simulink model "gm_flyback_pid"  (R2021b)
settings: Solver=FixedStepDiscrete  StartTime=0.0  StopTime=100e-3  RelTol=1e-3
undefined symbols (not defined in the file or in its folder): DiscIntNeverNeededParam
Description:
  | Symmetric FIR Filter
  | This example shows how to use HDL Coder(TM) to check, generate,
  | and verify HDL for a fixed-point symmetric FIR filter.
settings Model: Creator=The MathWorks, Inc.  LastModifiedBy=Marco Milanesi
settings SolverCC: AlgebraicLoopSolver=TrustRegion  AutoInsertRateTranBlk=on
settings DataIOCC: LimitDataPoints=on  SaveFormat=Array  SaveOutput=off  SignalLogging=off  SaveTime=off  ReturnWorkspaceOutputs=off  SignalLoggingName=logsOut
settings OptimizationCC: BlockReduction=off  BooleanDataType=off  ConditionallyExecuteInputs=off  DefaultParameterBehavior=Inlined  InheritOutputTypeSmallerThanSingle=on  InlineInvariantSignals=on  ExpressionDepthLimit=2147483647  InitFltsAndDblsToZero=on  LifeSpan=inf  BufferReusableBoundary=off
settings DebuggingCC: AlgebraicLoopMsg=error  SaveWithParameterizedLinksMsg=none  UnderspecifiedInitializationDetection=Classic  MergeDetectMultiDrivingBlocksExec=none  CheckExecutionContextPreStartOutputMsg=on  SignalResolutionControl=TryResolveAllWithWarning  InheritedTsInSrcMsg=none  MultiTaskDSMMsg=warning  MultiTaskCondExecSysMsg=none  SingleTaskRateTransMsg=error  IntegerOverflowMsg=none  ParameterPrecisionLossMsg=none  FcnCallInpInsideContextMsg=warning  BusObjectLabelMismatch=none  StateNameClashWarn=warning  SFUnexpectedBacktrackingDiag=warning  SFNoUnconditionalDefaultTransitionDiag=warning  SFExecutionAtInitializationDiag=none  SFMachineParentedDataDiag=warning  IntegerSaturationMsg=none  ArithmeticOperatorsInVariantConditions=warning
settings HardwareCC: ProdBitPerPointer=32  ProdBitPerSizeT=32  ProdBitPerPtrDiffT=32  ProdLargestAtomicFloat=None  ProdIntDivRoundTo=Undefined  ProdEndianess=Unspecified  ProdWordSize=32  ProdHWDeviceType=ASIC/FPGA  TargetUnknown=on  ProdEqTarget=off
settings ModelReferenceCC: PropagateSignalLabelsOutOfModel=off
settings SFSimCC: SimUseLocalCustomCode=off  CustomCodeUndefinedFunction=UseInterfaceOnly
settings RTWCC: RTWUseLocalCustomCode=off
settings CodeAppCC: StateflowObjectComments=on
settings GRTTargetCC: TargetFcnLib=ansi_tfl_tmw.mat  TargetLangStandard=C89/C90 (ANSI)  CombineOutputUpdateFcns=off  GRTInterface=on
settings ConfigComp: CovMetricSettings=dw  CovSaveCumulativeToWorkspaceVar=on  CovSaveSingleToWorkspaceVar=on  CovExternalEMLEnable=off

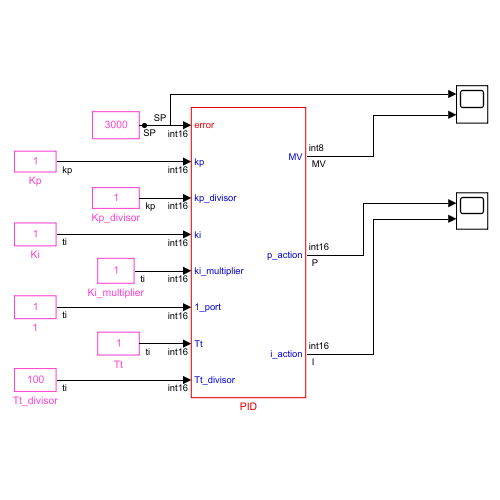
[thumbnail: Simulink's stored preview of the top-level diagram]
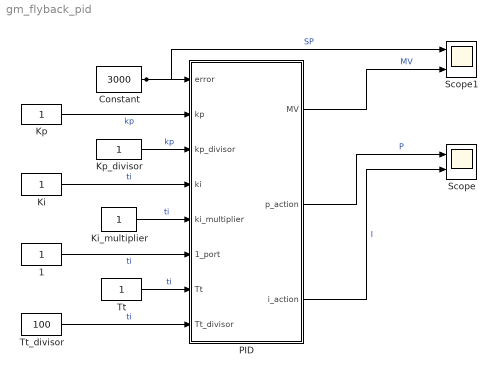
== system gm_flyback_pid ==
  1 : Constant  OutDataTypeStr=fixdt(1,16,0)
  Constant : Constant  Value=3000  OutDataTypeStr=fixdt(1,16,0)
  Ki : Constant  OutDataTypeStr=fixdt(1,16,0)
  Ki_multiplier : Constant  OutDataTypeStr=fixdt(1,16,0)
  Kp : Constant  OutDataTypeStr=fixdt(1,16,0)
  Kp_divisor : Constant  OutDataTypeStr=fixdt(1,16,0)
  PID : Subsystem
  Scope : Scope  NumInputPorts=2
  Scope1 : Scope  NumInputPorts=2
  Tt : Constant  OutDataTypeStr=fixdt(1,16,0)
  Tt_divisor : Constant  Value=100  OutDataTypeStr=fixdt(1,16,0)
  wires:
  Tt_divisor/1 -> PID/8(Tt_divisor)  "ti"
  Tt/1 -> PID/7(Tt)  "ti"
  1/1 -> PID/6(1_port)  "ti"
  Ki_multiplier/1 -> PID/5(ki_multiplier)  "ti"
  Kp_divisor/1 -> PID/3(kp_divisor)  "kp"
  PID/3(i_action) -> Scope/2  "I"
  PID/1(MV) -> Scope1/2  "MV"
  PID/2(p_action) -> Scope/1  "P"
  Constant/1 -> PID/1(error), Scope1/1  "SP"
  Ki/1 -> PID/4(ki)  "ti"
  Kp/1 -> PID/2(kp)  "kp"

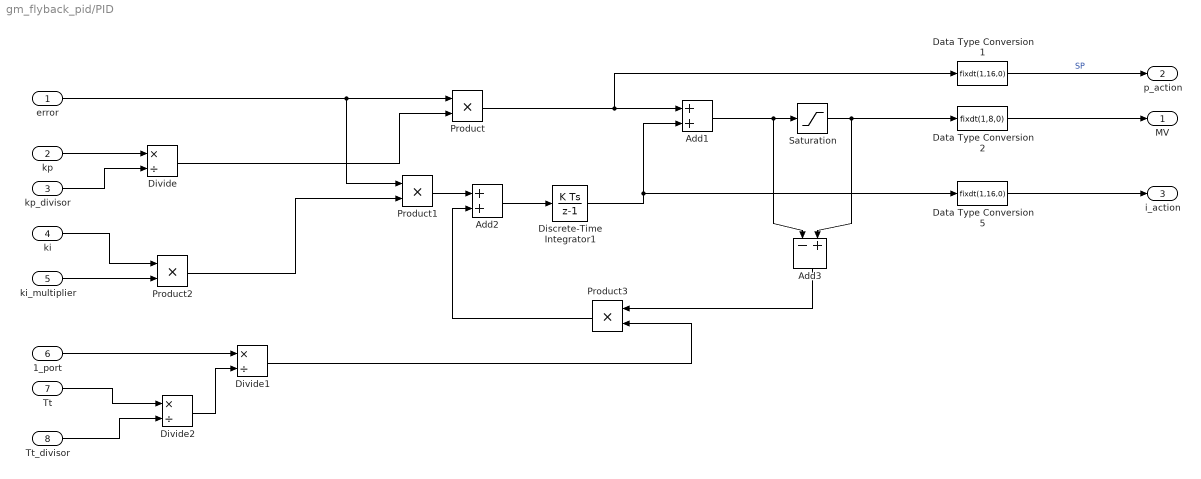
== system gm_flyback_pid/PID ==
  error : Inport  OutDataTypeStr=fixdt(1,16,0)  SampleTime=80e-9
  kp : Inport  Port=2  OutDataTypeStr=fixdt(1,16,0)  SampleTime=80e-9
  kp_divisor : Inport  Port=3  OutDataTypeStr=fixdt(1,16,0)  SampleTime=80e-9
  ki : Inport  Port=4  OutDataTypeStr=fixdt(1,16,0)  SampleTime=80e-9
  ki_multiplier : Inport  Port=5  OutDataTypeStr=fixdt(1,16,0)  SampleTime=80e-9
  1_port : Inport  Port=6  OutDataTypeStr=fixdt(1,16,0)  SampleTime=80e-9
  Tt : Inport  Port=7  OutDataTypeStr=fixdt(1,16,0)  SampleTime=80e-9
  Tt_divisor : Inport  Port=8  OutDataTypeStr=fixdt(1,16,0)  SampleTime=80e-9
  Add1 : Sum  AccumDataTypeStr=fixdt(1,16,0)  OutDataTypeStr=fixdt(1,16,0)
  Add2 : Sum  AccumDataTypeStr=fixdt(1,16,0)  OutDataTypeStr=fixdt(1,16,0)
  Add3 : Sum  Inputs=-+  AccumDataTypeStr=fixdt(1,16,0)  OutDataTypeStr=fixdt(1,16,0)
  Data Type Conversion1 : DataTypeConversion  OutDataTypeStr=fixdt(1,16,0)
  Data Type Conversion2 : DataTypeConversion  OutDataTypeStr=fixdt(1,8,0)
  Data Type Conversion5 : DataTypeConversion  OutDataTypeStr=fixdt(1,16,0)
  Discrete-Time Integrator1 : DiscreteIntegrator  SampleTime=80e-9  OutDataTypeStr=fixdt(1,16,0)  ICPrevOutput=DiscIntNeverNeededParam  ICPrevScaledInput=DiscIntNeverNeededParam
  Divide : Product  Inputs=*/  OutDataTypeStr=fixdt(1,16,0)  RndMeth=Zero  SaturateOnIntegerOverflow=on
  Divide1 : Product  Inputs=*/  OutDataTypeStr=fixdt(1,16,0)  RndMeth=Zero  SaturateOnIntegerOverflow=on
  Divide2 : Product  Inputs=*/  OutDataTypeStr=fixdt(1,16,0)  RndMeth=Zero  SaturateOnIntegerOverflow=on
  Product{,1..3} (4 alike) : Product  OutDataTypeStr=fixdt(1,16,0)
  Saturation : Saturate  UpperLimit=255  LowerLimit=0  OutDataTypeStr=fixdt(1,16,0)
  MV : Outport  OutDataTypeStr=fixdt(1,8,0)  SampleTime=80e-9  VectorParamsAs1DForOutWhenUnconnected=off
  p_action : Outport  Port=2  OutDataTypeStr=fixdt(1,16,0)  SampleTime=80e-9  VectorParamsAs1DForOutWhenUnconnected=off
  i_action : Outport  Port=3  OutDataTypeStr=fixdt(1,16,0)  SampleTime=80e-9  VectorParamsAs1DForOutWhenUnconnected=off
  wires:
  Divide2/1 -> Divide1/2
  1_port/1 -> Divide1/1
  Tt/1 -> Divide2/1
  Tt_divisor/1 -> Divide2/2
  Divide1/1 -> Product3/2
  Add2/1 -> Discrete-Time Integrator1/1
  Product1/1 -> Add2/1
  Add3/1 -> Product3/1
  Product3/1 -> Add2/2
  Add1/1 -> Add3/1, Saturation/1
  Saturation/1 -> Data Type Conversion2/1, Add3/2
  Product2/1 -> Product1/2
  ki/1 -> Product2/1
  ki_multiplier/1 -> Product2/2
  Divide/1 -> Product/2
  kp_divisor/1 -> Divide/2
  kp/1 -> Divide/1
  Data Type Conversion2/1 -> MV/1
  Data Type Conversion5/1 -> i_action/1
  Data Type Conversion1/1 -> p_action/1  "SP"
  Discrete-Time Integrator1/1 -> Add1/2, Data Type Conversion5/1
  Product/1 -> Add1/1, Data Type Conversion1/1
  error/1 -> Product1/1, Product/1
